simulink model "model"  (R2024b)
settings: Solver=VariableStepAuto  StartTime=0.0  StopTime=60  RelTol=1e-3
values from neighbouring files (symbols this model uses):
  initial_theta1 = alpha(i) + perturbed_theta1    [script.m]
  initial_theta2 = perturbed_theta2    (= 0.4)    [script.m]
settings Model: Creator=inarm  LastModifiedBy=plete
settings RTWCC: GPUComputeCapability=3.5

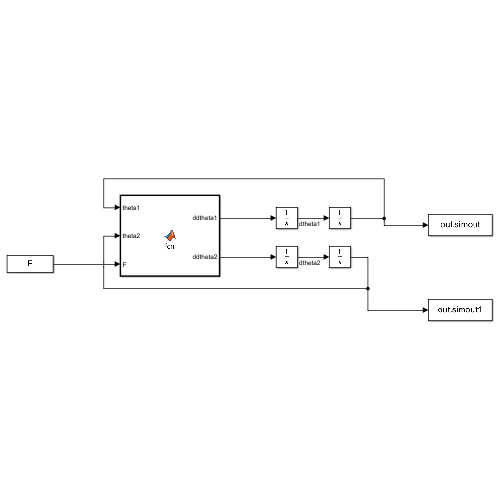
[thumbnail: Simulink's stored preview of the top-level diagram]
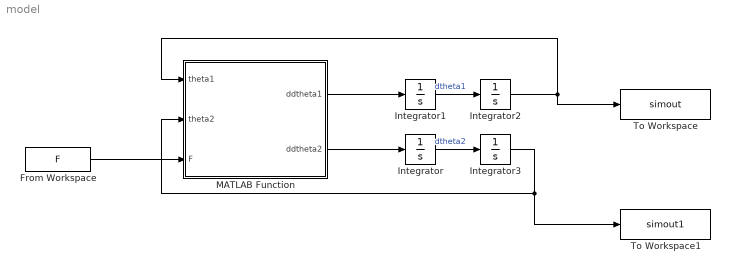
== system model ==
  From Workspace : FromWorkspace  VariableName=F
  Integrator : Integrator
  Integrator1 : Integrator
  Integrator2 : Integrator  InitialCondition=initial_theta1
  Integrator3 : Integrator  InitialCondition=initial_theta2
  MATLAB Function : MATLAB Function  TreatAsAtomicUnit=on
  To Workspace : ToWorkspace  VariableName=simout  SaveFormat=Timeseries  SampleTime=-1
  To Workspace1 : ToWorkspace  VariableName=simout1  SaveFormat=Timeseries  SampleTime=-1
  wires:
  MATLAB Function/2(ddtheta2) -> Integrator/1
  MATLAB Function/1(ddtheta1) -> Integrator1/1
  From Workspace/1 -> MATLAB Function/3(F)
  Integrator/1 -> Integrator3/1  "dtheta2"
  Integrator1/1 -> Integrator2/1  "dtheta1"
  Integrator2/1 -> To Workspace/1, MATLAB Function/1(theta1)
  Integrator3/1 -> To Workspace1/1, MATLAB Function/2(theta2)

== matlab function model/MATLAB Function ==
  data: theta1 input; ddtheta1 output; theta2 input; F input; ddtheta2 output
function [ddtheta1, ddtheta2] = fcn(theta1,theta2,F)

M = 2;
L = 1;
g = 10;
k = 1;

sin_theta1 = sin(theta1);
sin_theta2 = sin(theta2);
cos_theta1 = cos(theta1);
cos_theta2 = cos(theta2);

ddtheta1 = (F - M*g*L*sin_theta1 - (1/4)*k*L^2*(sin_theta1 - sin_theta2)*cos_theta1) / (M*L^2);

ddtheta2 = (- M*g*L*sin_theta2 + (1/4)*k*L^2*(sin_theta1 - sin_theta2)*cos_theta2) / (M*L^2);
